simulink library "Aero_Lib"  (Simulink 8.0)
settings: Solver=ode45  StartTime=0.0  StopTime=10.0  RelTol=1e-3
values from neighbouring files (symbols this model uses):
  AC = miniMUTT_config    [UAV_config.m]    (also in UAV_modelconfig.mat = )
libraries: UltraStick120_Aero_Lib x2, UltraStick25e_Aero_Lib x2, Aero_Lib x1, simulink x1, aerolibadyn x1, miniMUTT_Aero_Lib x1
settings Model: Creator=austinmurch  LastModifiedBy=brtaylor

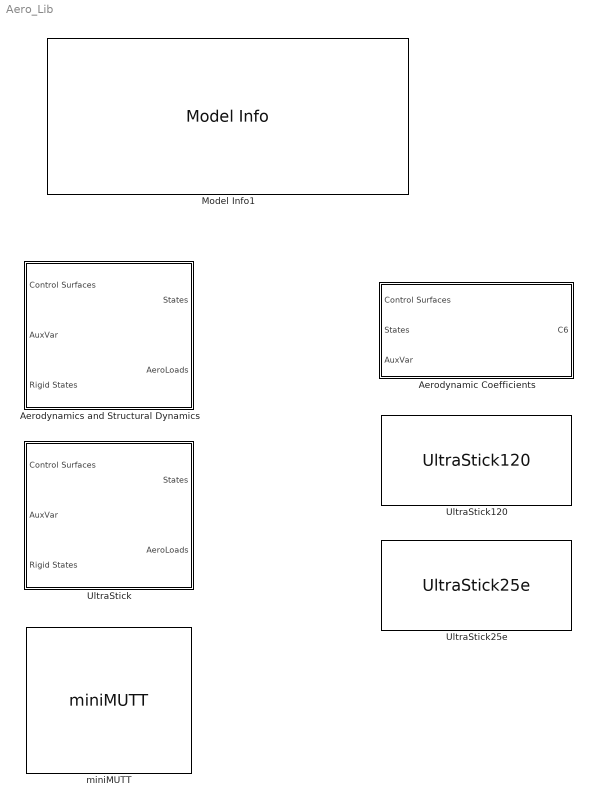
== system Aero_Lib ==
  Aerodynamic Coefficients : Subsystem  BlockChoice=UltraStick120
      settings: TemplateBlock=self  MemberBlocks=UltraStick120,UltraStick25e
  Aerodynamics and Structural Dynamics : Subsystem  BlockChoice=UltraStick  mask{aircraft=AC.aircraft}
      mask prompts: aircraft "Aircraft Type:"
      mask help: Select aerodynamic model based on AC.aircraft variable
      mask init:
      | pathname = gcb;
      | 
      | switch lower(aircraft)
      |     case 'ultrastick120'
      |         set_param(pathname,'BlockChoice','UltraStick');
      |         set_param([pathname '/UltraStick/Aerodynamic Coefficients'],'BlockChoice','UltraStick120');
      | %         set_param([pathname '/UltraStick/Forces and Moments Calculation'],'inputAxes','Stability');
      | %         set_param([pathname '/UltraStick/Forces and Moments Calculation'],'outputMomentAxes','Stability');
      |     case 'ultrastick25e'
      |         set_param(pathname,'BlockChoice','UltraStick');
      |         set_param([pathname '/UltraStick/Aerodynamic Coefficients'],'BlockChoice','UltraStick25e');
      | %         set_param([pathname '/UltraStick/Forces and Moments Calculation'],'inputAxes','Wind');
      | %         set_param([pathname '/UltraStick/Forces and Moments Calculation'],'outputMomentAxes','Wind');
      |     case 'minimutt'
      |         set_param(pathname,'BlockChoice','miniMUTT');
      | end
      settings: TemplateBlock=self  MemberBlocks=UltraStick,miniMUTT
  Model Info1 : simulink/Model-Wide Utilities/Model Info  InitialBlockCM=None  BlockCM=None  Frame=on  DisplayStringWithTags=|  HorizontalTextAlignment=Left  LeftAlignmentValue=0.02  SourceBlockDiagram=Aero_Lib  TagMaxNumber=20
      | MODEL INFORMATION
      | Aerodynamic Model Library
      | 
      | University of Minnesota
      | Aerospace Engineering and Mechanics
      | Copyright 2011 Regents of the University of Minnesota. All rights reserved.
      | 
      | == SVN Info ==
      | Last modified by %<LastModifiedBy> on %<LastModificationDate>
  UltraStick : Subsystem  mask{aircraft=AC.aircraft}
      mask prompts: aircraft "Aircraft Type:"
      mask init:
      | pathname = gcb;
      | 
      | switch lower(aircraft)
      |     case 'ultrastick120'
      |         set_param([pathname '/Forces and Moments Calculation'],'inputAxes','Stability');
      |         set_param([pathname '/Forces and Moments Calculation'],'outputMomentAxes','Stability');
      |     case 'ultrastick25e'
      |         set_param([pathname '/Forces and Moments Calculation'],'inputAxes','Wind');
      |         set_param([pathname '/Forces and Moments Calculation'],'outputMomentAxes','Wind');
      | end
  UltraStick120 : UltraStick120_Aero_Lib/UltraStick120
  UltraStick25e : UltraStick25e_Aero_Lib/UltraStick25e
  miniMUTT : miniMUTT_Aero_Lib/miniMUTT

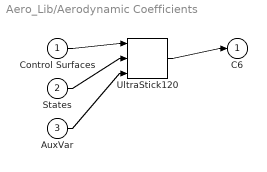
== system Aero_Lib/Aerodynamic Coefficients ==
  Control Surfaces : Inport
  States : Inport  Port=2
  AuxVar : Inport  Port=3
  UltraStick120 : UltraStick120_Aero_Lib/UltraStick120
  C6 : Outport
  wires:
  Control Surfaces/1 -> UltraStick120/1
  States/1 -> UltraStick120/2
  AuxVar/1 -> UltraStick120/3
  UltraStick120/1 -> C6/1

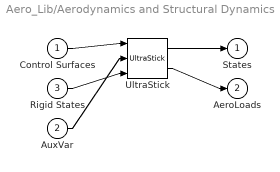
== system Aero_Lib/Aerodynamics and Structural Dynamics ==
  Control Surfaces : Inport
  AuxVar : Inport  Port=2
  Rigid States : Inport  Port=3
  UltraStick : Aero_Lib/UltraStick  aircraft=AC.aircraft
      link override Aerodynamic Coefficients: BlockChoice=UltraStick25e
  States : Outport
  AeroLoads : Outport  Port=2
  wires:
  Control Surfaces/1 -> UltraStick/1
  AuxVar/1 -> UltraStick/2
  Rigid States/1 -> UltraStick/3
  UltraStick/1 -> States/1
  UltraStick/2 -> AeroLoads/1

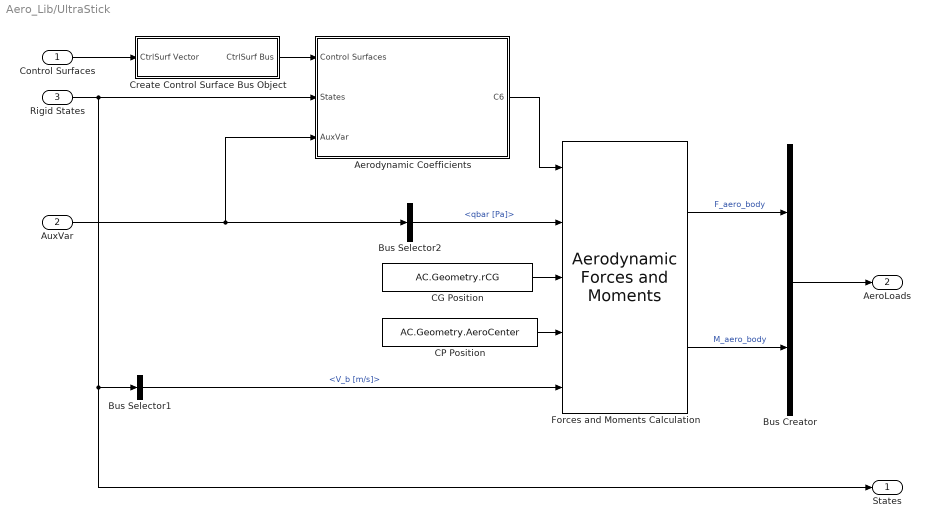
== system Aero_Lib/UltraStick ==
  Control Surfaces : Inport
  AuxVar : Inport  Port=2
  Rigid States : Inport  Port=3
  Aerodynamic Coefficients : Subsystem  BlockChoice=UltraStick25e
      settings: AttributesFormatString=%<BlockChoice>  TemplateBlock=Aero_Lib/Aerodynamic Coefficients  MemberBlocks=UltraStick120,UltraStick25e
  Bus Selector1 : BusSelector  OutputSignals=V_b [m/s]
  Bus Creator : BusCreator  Inputs=2
  Bus Selector2 : BusSelector  OutputSignals=qbar [Pa]
  CG Position : Constant  Value=AC.Geometry.rCG
  CP Position : Constant  Value=AC.Geometry.AeroCenter
  Create Control Surface Bus Object : Subsystem
  Forces and Moments Calculation : aerolibadyn/Aerodynamic Forces and Moments   inputAxes=Wind  outputForceAxes=Body  outputMomentAxes=Wind  S=AC.Geometry.S  b=AC.Geometry.b  cbar=AC.Geometry.c
  States : Outport
  AeroLoads : Outport  Port=2
  wires:
  Bus Selector1/1 -> Forces and Moments Calculation/5  "<V_b [m/s]>"
  CG Position/1 -> Forces and Moments Calculation/3
  CP Position/1 -> Forces and Moments Calculation/4
  Rigid States/1 -> States/1, Bus Selector1/1, Aerodynamic Coefficients/2(States)
  Forces and Moments Calculation/1 -> Bus Creator/1  "F_aero_body"
  Control Surfaces/1 -> Create Control Surface Bus Object/1(CtrlSurf Vector)
  Bus Creator/1 -> AeroLoads/1
  Forces and Moments Calculation/2 -> Bus Creator/2  "M_aero_body"
  AuxVar/1 -> Aerodynamic Coefficients/3(AuxVar), Bus Selector2/1
  Bus Selector2/1 -> Forces and Moments Calculation/2  "<qbar [Pa]>"
  Aerodynamic Coefficients/1(C6) -> Forces and Moments Calculation/1
  Create Control Surface Bus Object/1(CtrlSurf Bus) -> Aerodynamic Coefficients/1(Control Surfaces)

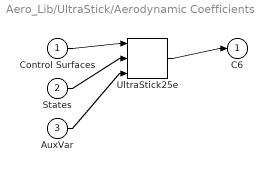
== system Aero_Lib/UltraStick/Aerodynamic Coefficients ==
  Control Surfaces : Inport
  States : Inport  Port=2
  AuxVar : Inport  Port=3
  UltraStick25e : UltraStick25e_Aero_Lib/UltraStick25e
  C6 : Outport
  wires:
  Control Surfaces/1 -> UltraStick25e/1
  States/1 -> UltraStick25e/2
  AuxVar/1 -> UltraStick25e/3
  UltraStick25e/1 -> C6/1

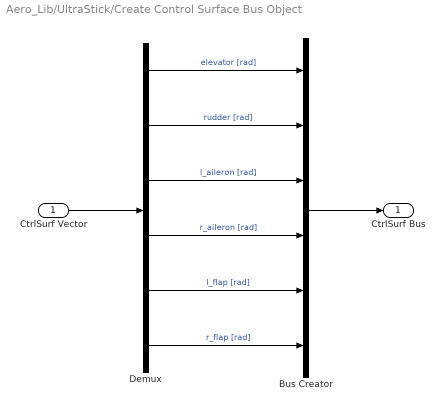
== system Aero_Lib/UltraStick/Create Control Surface Bus Object ==
  CtrlSurf Vector : Inport
  Bus Creator : BusCreator  Inputs=6
  Demux : Demux  Outputs=6
  CtrlSurf Bus : Outport
  wires:
  CtrlSurf Vector/1 -> Demux/1
  Demux/6 -> Bus Creator/6  "r_flap [rad]"
  Demux/3 -> Bus Creator/3  "l_aileron [rad]"
  Demux/4 -> Bus Creator/4  "r_aileron [rad]"
  Demux/2 -> Bus Creator/2  "rudder [rad]"
  Demux/1 -> Bus Creator/1  "elevator [rad]"
  Demux/5 -> Bus Creator/5  "l_flap [rad]"
  Bus Creator/1 -> CtrlSurf Bus/1
